simulink model "myFirstRelayWithThreeOutputsModel"  (R2022a)
settings: Solver=VariableStepAuto  StartTime=0.0  StopTime=H-1  RelTol=1e-3
values from neighbouring files (symbols this model uses):
  eps1 = 2    [myFirstRelayWithThreeOutputs.m]
  eps2 = -2    [myFirstRelayWithThreeOutputs.m]
  q_star = 1000    [init.m]    (also in myFirstRelayWithThreeOutputs.m = 10)
settings Model: Creator=mrnel  LastModifiedBy=mrnel

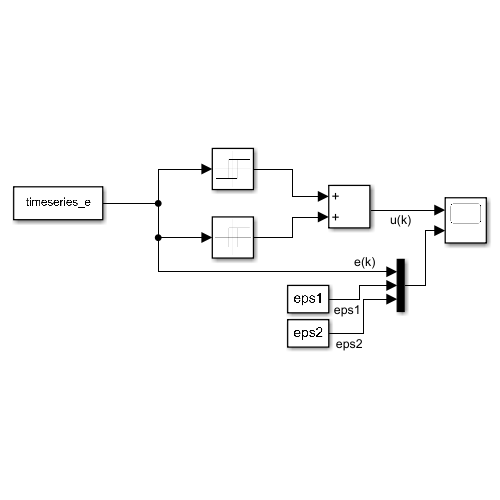
[thumbnail: Simulink's stored preview of the top-level diagram]
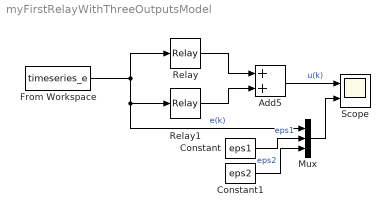
== system myFirstRelayWithThreeOutputsModel ==
  Add5 : Sum
  Constant : Constant  Value=eps1
  Constant1 : Constant  Value=eps2
  From Workspace : FromWorkspace  VariableName=timeseries_e
  Mux : Mux  Inputs=3
  Relay : Relay  OnSwitchValue=eps1  OffSwitchValue=eps1  OnOutputValue=-q_star/2  OffOutputValue=q_star/2
  Relay1 : Relay  OnSwitchValue=eps2  OffSwitchValue=eps2  OnOutputValue=-q_star/2  OffOutputValue=q_star/2
  Scope : Scope  NumInputPorts=2
  wires:
  Add5/1 -> Scope/1  "u(k)"
  Relay/1 -> Add5/1
  Relay1/1 -> Add5/2
  Constant/1 -> Mux/2  "eps1"
  From Workspace/1 -> Relay/1, Mux/1, Relay1/1  "e(k)"
  Constant1/1 -> Mux/3  "eps2"
  Mux/1 -> Scope/2
